simulink model "wykresy"  (R2019b)
settings: Solver=ode45  StartTime=0.0  StopTime=10.0  MaxStep=0.05  RelTol=1e-3  AbsTol=1e-6  EnableMultiTasking=on
values from neighbouring files (symbols this model uses):
  A1 = 1    [Lab06.m]
  a1 = (Aw1.*sqrt(2.*g.*h1max))/(h1max)    [Lab06.m]
  A2 = 2    [Lab06.m]
  a2 = (Aw2.*sqrt(2.*g.*h2max))/(h2max)    [Lab06.m]
  dfwe1 = 0    [Lab06.m]
  dfwe2 = 0.1*fwe2max    [Lab06.m]
  fwe1 = 0.2.*fwe1max    [Lab06.m]
  fwe2 = fwe2tab(i)    [Lab06.m]
  h01 = fwe1./a1    [Lab06.m]
  h02 = (fwe2+fwe1)./a2    [Lab06.m]
  t0 = 2    [Lab06.m]
settings Model: Creator=LAB320-1552  LastModifiedBy=Gabriel Mainka
settings SolverCC: AutoScaleAbsTol=off
settings DataIOCC: LimitDataPoints=on  SaveFormat=Array  ReturnWorkspaceOutputs=off
settings OptimizationCC: LifeSpan=inf
settings DebuggingCC: UnderspecifiedInitializationDetection=Classic  MergeDetectMultiDrivingBlocksExec=none  StateNameClashWarn=warning  SFUnexpectedBacktrackingDiag=warning  SFNoUnconditionalDefaultTransitionDiag=warning  SFExecutionAtInitializationDiag=none  ArithmeticOperatorsInVariantConditions=warning
settings HardwareCC: ProdBitPerPointer=32  ProdBitPerSizeT=32  ProdBitPerPtrDiffT=32  ProdLargestAtomicFloat=None  ProdIntDivRoundTo=Undefined  ProdEndianess=Unspecified  ProdWordSize=32  ProdHWDeviceType=32-bit Generic
settings ModelReferenceCC: PropagateSignalLabelsOutOfModel=off
settings SFSimCC: SimUseLocalCustomCode=off  CustomCodeUndefinedFunction=UseInterfaceOnly
settings RTWCC: RTWUseLocalCustomCode=off
settings CodeAppCC: StateflowObjectComments=on
settings GRTTargetCC: TargetLangStandard=C89/C90 (ANSI)  GeneratePreprocessorConditionals=Disable all
settings ConfigComp: CovMetricSettings=dw  CovHtmlReporting=on  CovSaveCumulativeToWorkspaceVar=on  CovSaveSingleToWorkspaceVar=on  CovExternalEMLEnable=off

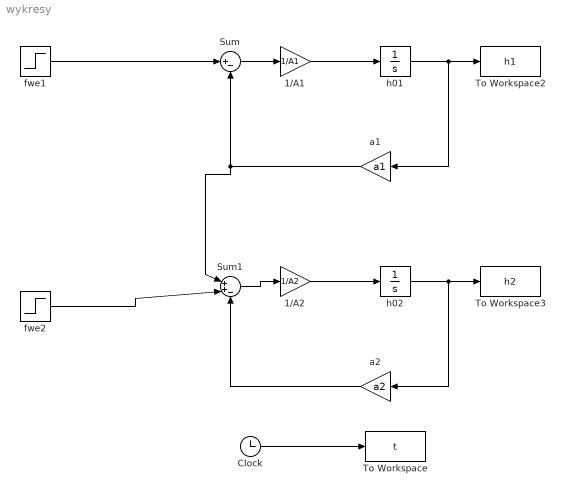
== system wykresy ==
  1/A1 : Gain  Gain=1/A1
  1/A2 : Gain  Gain=1/A2
  Clock : Clock
  Sum : Sum  Inputs=|+-
  Sum1 : Sum  Inputs=|++-
  To Workspace : ToWorkspace  VariableName=t  SampleTime=-1
  To Workspace2 : ToWorkspace  VariableName=h1  SampleTime=-1
  To Workspace3 : ToWorkspace  VariableName=h2  SampleTime=-1
  a1 : Gain  Gain=a1
  a2 : Gain  Gain=a2
  fwe1 : Step  Time=t0  Before=fwe1  After=fwe1+dfwe1  SampleTime=0
  fwe2 : Step  Time=t0  Before=fwe2  After=fwe2+dfwe2  SampleTime=0
  h01 : Integrator  InitialCondition=h01
  h02 : Integrator  InitialCondition=h02
  wires:
  Clock/1 -> To Workspace/1
  fwe1/1 -> Sum/1
  Sum/1 -> 1/A1/1
  1/A1/1 -> h01/1
  h01/1 -> a1/1, To Workspace2/1
  a1/1 -> Sum/2, Sum1/1
  Sum1/1 -> 1/A2/1
  1/A2/1 -> h02/1
  h02/1 -> a2/1, To Workspace3/1
  fwe2/1 -> Sum1/2
  a2/1 -> Sum1/3
